simulink model "Ilagan_Arcega_SIMULINK_LAB3_ReducedBlockDiagram_No1"  (R2024a)
settings: Solver=VariableStepAuto  StartTime=0.0  StopTime=20.0  RelTol=1e-3
values from neighbouring files (symbols this model uses):
  TF_den = conv(TF4_den,TF6_den)    [Ilagan_Arcega_LAB3_ReducedBlockDiagram_No1.m]
  TF_num = conv(TF4_num,TF6_num)    [Ilagan_Arcega_LAB3_ReducedBlockDiagram_No1.m]
settings Model: Creator=Kyla Ilagan  LastModifiedBy=Kyla Ilagan

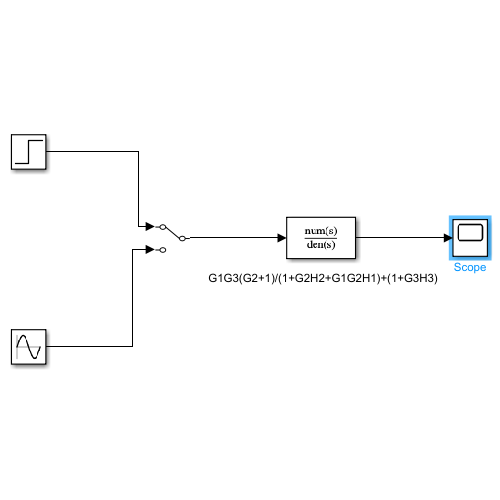
[thumbnail: Simulink's stored preview of the top-level diagram]
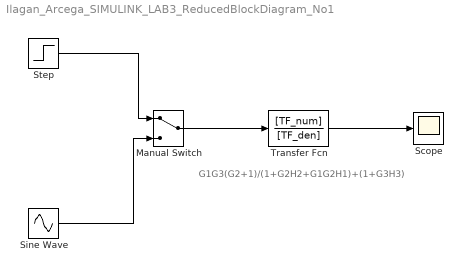
== system Ilagan_Arcega_SIMULINK_LAB3_ReducedBlockDiagram_No1 ==
  note: G1G3(G2+1)/(1+G2H2+G1G2H1)+(1+G3H3)
  Manual Switch : ManualSwitch
  Scope : Scope
  Sine Wave : Sin  SampleTime=0
  Step : Step  SampleTime=0
  Transfer Fcn : TransferFcn  Numerator=[TF_num]  Denominator=[TF_den]
  wires:
  Step/1 -> Manual Switch/1
  Sine Wave/1 -> Manual Switch/2
  Manual Switch/1 -> Transfer Fcn/1
  Transfer Fcn/1 -> Scope/1
